simulink model "RLTunningTV"  (R2019b)
settings: Solver=odeN  StartTime=0.0  StopTime=15  FixedStep=0.001  RelTol=1e-3
PreLoadFcn:
  | Vehicle_parameters;
  | hcc_init;
InitFcn:
  | Vehicle_parameters;
  | hcc_init;
values from neighbouring files (symbols this model uses):
  c = (1.596+1.610)/2    (= 1.603)    [Vehicle_parameters.m]
  g = 9.8    [Vehicle_parameters.m]
  gamma = 0.006    [hcc_init.m]
  Jzz = 2050    [Vehicle_parameters.m]
  kx1 = 0.05890269    [hcc_init.m]
  ky1 = 0.04086363    [hcc_init.m]
  kz1 = 0.27516026    [hcc_init.m]
  lf = 1.3265    [Vehicle_parameters.m]
  lr = 1.3685    [Vehicle_parameters.m]
  M = 1360    [Vehicle_parameters.m]
  n = 6    [hcc_init.m]    (also in smoothing_t0.m = 16)
  pbk_gain = 1.0    (= 1)    [hcc_init.m]
  Q_gain = 50.0    (= 50)    [hcc_init.m]
  Qf = [0.0, 0.0 ... (first row only)    [hcc_init.m]
  Qr = [0.0, 0.0 ... (first row only)    [hcc_init.m]
  Reff = 0.323    [Vehicle_parameters.m]
  swa_gain = 45.0    (= 45)    [hcc_init.m]
  umax_m = 4000.0    (= 4000)    [hcc_init.m]
  umin_br = umin_m + umin_b    (= -4500)    [hcc_init.m]
  v = 80    [Vehicle_parameters.m]
  wFx = 0.4    [hcc_init.m]
  wFy = 0.02    [hcc_init.m]
  wGz = 1500.89459504    [hcc_init.m]
undefined symbols (not defined in the file or in its folder): DiscIntNeverNeededParam, LMUX, LMUY, sigbuilder_block
libraries: simulink x10, rllib x1
(part 1 of 3)
settings Model: Creator=st00853  LastModifiedBy=st00853
settings SolverCC: ZeroCrossControl=DisableAll
settings DebuggingCC: ArithmeticOperatorsInVariantConditions=warning
settings SFSimCC: CustomCodeUndefinedFunction=UseInterfaceOnly

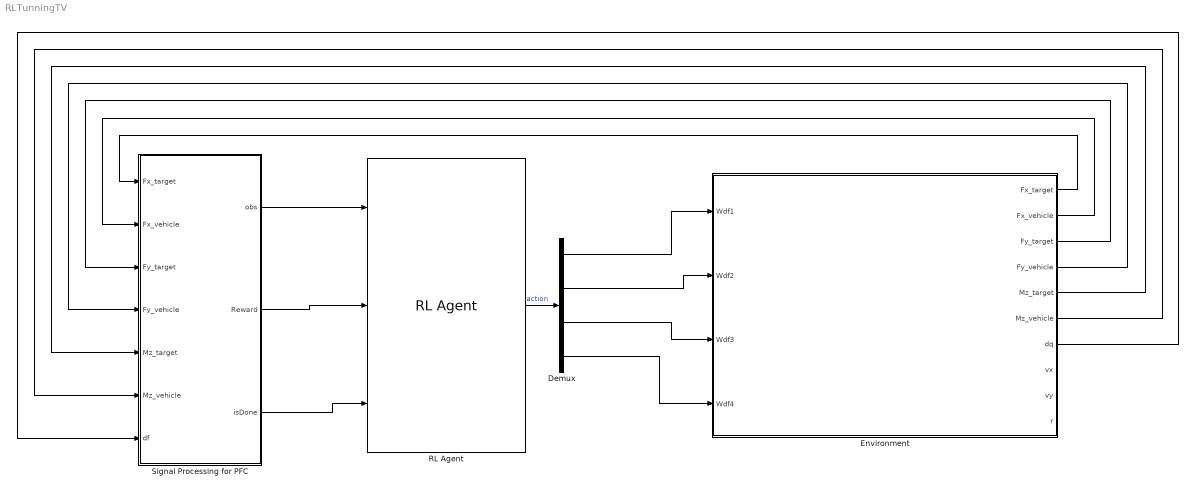
== system RLTunningTV ==
  Demux : Demux
  Environment : Subsystem
  RL Agent : rllib/RL Agent  Agent=agent  ProvideReward=on  ProvideIsDone=on  ProvideCumRwd=off  TreatAsDirectFeedthrough=on  CollectLoggedSignals=on  CollectModelStates=on
      settings: SourceProductName=Reinforcement Learning Toolbox
  Signal Processing for PFC : Subsystem
  wires:
  RL Agent/1 -> Demux/1  "action"
  Demux/1 -> Environment/1(Wdf1)
  Demux/2 -> Environment/2(Wdf2)
  Demux/3 -> Environment/3(Wdf3)
  Demux/4 -> Environment/4(Wdf4)
  Signal Processing for PFC/2(Reward) -> RL Agent/2
  Signal Processing for PFC/1(obs) -> RL Agent/1
  Signal Processing for PFC/3(isDone) -> RL Agent/3
  Environment/7(dq) -> Signal Processing for PFC/7(df)
  Environment/1(Fx_target) -> Signal Processing for PFC/1(Fx_target)
  Environment/2(Fx_vehicle) -> Signal Processing for PFC/2(Fx_vehicle)
  Environment/3(Fy_target) -> Signal Processing for PFC/3(Fy_target)
  Environment/4(Fy_vehicle) -> Signal Processing for PFC/4(Fy_vehicle)
  Environment/6(Mz_vehicle) -> Signal Processing for PFC/6(Mz_vehicle)
  Environment/5(Mz_target) -> Signal Processing for PFC/5(Mz_target)

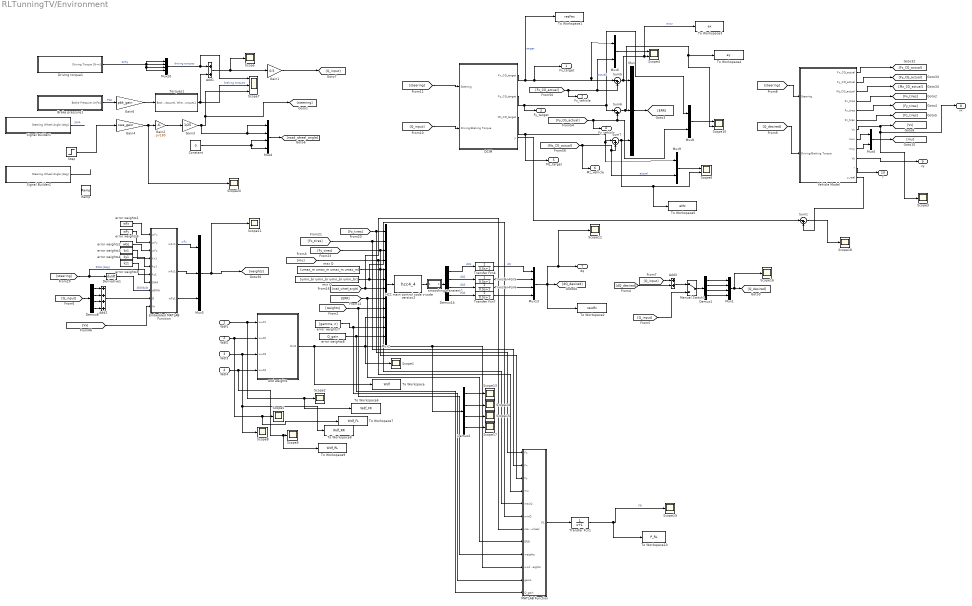
== system RLTunningTV/Environment ==
  Wdf1 : Inport
  Wdf2 : Inport  Port=2
  Wdf3 : Inport  Port=3
  Wdf4 : Inport  Port=4
  Add1 : Sum
  Add2 : Sum  Inputs=++++
  Add3 : Sum
  Brake pressure1 : Subsystem  Tag=STV Subsys  LoadFcn=sigbuilder_block('load');  StartFcn=sigbuilder_block('start');  StopFcn=sigbuilder_block('stop');  ClipboardFcn=sigbuilder_block('clipboard');  mask(Sigbuilder block){tuvar=[0:10]}
      mask help: Sigbuilder GUI
      mask init:
      | if ~strcmp(get_param(bdroot(gcbh),'SimulationStatus'),'stopped') tuvar = sigbuilder_block('maskInit'); end
      settings: CopyFcn=sigbuilder_block('copy');  DeleteFcn=sigbuilder_block('delete');  ModelCloseFcn=sigbuilder_block('modelClose');  PreSaveFcn=sigbuilder_block('preSave');  PauseFcn=sigbuilder_block('pause')  ContinueFcn=sigbuilder_block('continue')  NameChangeFcn=sigbuilder_block('namechange');  OpenFcn=sigbuilder_block('open',[0 0 1131 540.75 ]);  CloseFcn=sigbuilder_block('close');
      mask Display: plot(0, 0, 100, 100,[2, 2, 32, 32, 2], [68, 8, 8, 68, 68],[32, 2], [38, 38], [32, 19, 2],[53, 60, 44], [32, 17, 17, 2],[16, 16, 31, 31]);txt = getActiveGroup(gcbh);text(2, 100, txt,'verticalAlignment', 'top');
  Constant : Constant  Value=0
  DCIM : Subsystem
  Demux{1..2,8,14} (4 alike) : Demux
  Derivative1 : Derivative
  Driving torque1 : Subsystem  Tag=STV Subsys  LoadFcn=sigbuilder_block('load');  StartFcn=sigbuilder_block('start');  StopFcn=sigbuilder_block('stop');  ClipboardFcn=sigbuilder_block('clipboard');  mask(Sigbuilder block){tuvar=[0:10]}
      mask help: Sigbuilder GUI
      mask init:
      | if ~strcmp(get_param(bdroot(gcbh),'SimulationStatus'),'stopped') tuvar = sigbuilder_block('maskInit'); end
      settings: CopyFcn=sigbuilder_block('copy');  DeleteFcn=sigbuilder_block('delete');  ModelCloseFcn=sigbuilder_block('modelClose');  PreSaveFcn=sigbuilder_block('preSave');  PauseFcn=sigbuilder_block('pause')  ContinueFcn=sigbuilder_block('continue')  NameChangeFcn=sigbuilder_block('namechange');  OpenFcn=sigbuilder_block('open',[0 0 1131 540.75 ]);  CloseFcn=sigbuilder_block('close');
      mask Display: plot(0, 0, 100, 100,[2, 2, 32, 32, 2], [68, 8, 8, 68, 68],[32, 2], [38, 38], [32, 19, 2],[53, 60, 44], [32, 17, 17, 2],[16, 16, 31, 31]);txt = getActiveGroup(gcbh);text(2, 100, txt,'verticalAlignment', 'top');
  Embedded MATLAB Function : MATLAB Function  TreatAsAtomicUnit=on
  Gain1 : Gain  Gain=0.5  SampleTime=0.001
  Gain2 : Gain  Gain=pi/180
  Gain3 : Gain  Gain=1/25  SampleTime=0.001
  Gain4 : Gain  Gain=swa_gain  SampleTime=0.001
  Gain6 : Gain  Gain=pbk_gain  SampleTime=0.001
  HCC main control code c-code version2 : S-Function  FunctionName=hcc4_4  SFunctionDeploymentMode=off  EnableBusSupport=off
  MATLAB Function : MATLAB Function  TreatAsAtomicUnit=on
  Manual Switch1 : ManualSwitch
  Mux : Mux  Inputs=3
  Mux{1,4,13,20} (4 alike) : Mux
  Mux2 : Mux  Inputs=12
  Mux3 : Mux  Inputs=3
  Mux{5..6,8..9} (4 alike) : Mux  Inputs=2
  Ramp : simulink/Sources/Ramp  slope=0.1  start=3  InitialOutput=0
  Scope{,1..3,5,8..9,11..20} (17 alike) : Scope
  Scope10 : Scope  NumInputPorts=2
  Scope4 : Scope  NumInputPorts=2
  Scope6 : Scope  NumInputPorts=2
  Scope7 : Scope  NumInputPorts=3
  Signal Builder1 : Subsystem  Tag=STV Subsys  LoadFcn=sigbuilder_block('load');  StartFcn=sigbuilder_block('start');  StopFcn=sigbuilder_block('stop');  ClipboardFcn=sigbuilder_block('clipboard');  mask(Sigbuilder block){tuvar=[0:10]}
      mask help: Sigbuilder GUI
      mask init:
      | if ~strcmp(get_param(bdroot(gcbh),'SimulationStatus'),'stopped') tuvar = sigbuilder_block('maskInit'); end
      settings: CopyFcn=sigbuilder_block('copy');  DeleteFcn=sigbuilder_block('delete');  ModelCloseFcn=sigbuilder_block('modelClose');  PreSaveFcn=sigbuilder_block('preSave');  PauseFcn=sigbuilder_block('pause')  ContinueFcn=sigbuilder_block('continue')  NameChangeFcn=sigbuilder_block('namechange');  OpenFcn=sigbuilder_block('open',[96.75 77.25 1131 540.75 ]);  CloseFcn=sigbuilder_block('close');
      mask Display: plot(0, 0, 100, 100,[2, 2, 32, 32, 2], [68, 8, 8, 68, 68],[32, 2], [38, 38], [32, 19, 2],[53, 60, 44], [32, 17, 17, 2],[16, 16, 31, 31]);txt = getActiveGroup(gcbh);text(2, 100, txt,'verticalAlignment', 'top');
  Signal Builder2 : Subsystem  Tag=STV Subsys  LoadFcn=sigbuilder_block('load');  StartFcn=sigbuilder_block('start');  StopFcn=sigbuilder_block('stop');  ClipboardFcn=sigbuilder_block('clipboard');  mask(Sigbuilder block){tuvar=[0:10]}
      mask help: Sigbuilder GUI
      mask init:
      | if ~strcmp(get_param(bdroot(gcbh),'SimulationStatus'),'stopped') tuvar = sigbuilder_block('maskInit'); end
      settings: CopyFcn=sigbuilder_block('copy');  DeleteFcn=sigbuilder_block('delete');  ModelCloseFcn=sigbuilder_block('modelClose');  PreSaveFcn=sigbuilder_block('preSave');  PauseFcn=sigbuilder_block('pause')  ContinueFcn=sigbuilder_block('continue')  NameChangeFcn=sigbuilder_block('namechange');  OpenFcn=sigbuilder_block('open',[111 159.75 1131 540.75 ]);  CloseFcn=sigbuilder_block('close');
      mask Display: plot(0, 0, 100, 100,[2, 2, 32, 32, 2], [68, 8, 8, 68, 68],[32, 2], [38, 38], [32, 19, 2],[53, 60, 44], [32, 17, 17, 2],[16, 16, 31, 31]);txt = getActiveGroup(gcbh);text(2, 100, txt,'verticalAlignment', 'top');
  Step : Step  Time=3.5  SampleTime=0.001
  Sum{1,5..7} (4 alike) : Sum  Inputs=|-+
  To Workspace : ToWorkspace  VariableName=Wdf  SaveFormat=Structure With Time  SampleTime=-1
  To Workspace1 : ToWorkspace  VariableName=resFex  SaveFormat=Structure With Time  SampleTime=-1
  To Workspace10 : ToWorkspace  VariableName=P_RL  SaveFormat=Structure With Time  SampleTime=-1
  To Workspace2 : ToWorkspace  VariableName=resdfx  SaveFormat=Structure With Time  SampleTime=-1
  To Workspace3 : ToWorkspace  VariableName=ex  SaveFormat=Structure With Time  SampleTime=-1
  To Workspace4 : ToWorkspace  VariableName=ey  SaveFormat=Structure With Time  SampleTime=-1
  To Workspace5 : ToWorkspace  VariableName=eMz  SaveFormat=Structure With Time  SampleTime=-1
  To Workspace6 : ToWorkspace  VariableName=Wdf_FR  SaveFormat=Structure With Time  SampleTime=-1
  To Workspace7 : ToWorkspace  VariableName=Wdf_FL  SaveFormat=Structure With Time  SampleTime=-1
  To Workspace8 : ToWorkspace  VariableName=Wdf_RR  SaveFormat=Structure With Time  SampleTime=-1
  To Workspace9 : ToWorkspace  VariableName=Wdf_RL  SaveFormat=Structure With Time  SampleTime=-1
  Torques1 : Subsystem
  Transfer Fcn1 : TransferFcn  Denominator=[1 1]
  Transfer Fcn{4..7} (4 alike) : TransferFcn  Denominator=[0.5 1]
  Vehicle Model : Subsystem
  error weights1 : Constant  Value=wFx
  error weights2 : Constant  Value=wGz
  error weights3 : Constant  Value=kx1
  error weights4 : Constant  Value=ky1
  error weights5 : Constant  Value=kz1
  error weights6 : Constant  Value=wFy
  error weights7 : Constant  Value=[gamma, n]
  error weights8 : Constant  Value=Q_gain
  max Q : Constant  Value=[umax_m umax_m umax_m umax_m]
  min Q : Constant  Value=[umin_br umin_br umin_br umin_br]
  smoothing transient2 : Subsystem
  wxd weights : Subsystem
  Fx_target : Outport
  Fx_vehicle : Outport  Port=2
  Fy_target : Outport  Port=3
  Fy_vehicle : Outport  Port=4
  Mz_target : Outport  Port=5
  Mz_vehicle : Outport  Port=6
  dq : Outport  Port=7
  vx : Outport  Port=8
  vy : Outport  Port=9
  r : Outport  Port=10
  wires:
  Demux1/3 -> Mux1/3
  Transfer Fcn6/1 -> Mux13/3
  Demux1/4 -> Mux1/4
  Vehicle Model/8(mux) -> Mux5/1
  Constant/1 -> Mux4/4, Mux4/3
  error weights3/1 -> Embedded MATLAB Function/4(kx1)
  Embedded MATLAB Function/1(wFx1) -> Mux3/1  "wFx"
  max Q/1 -> MATLAB Function/5(maxQ), Mux2/5
  Vehicle Model/3("Mz_CG_actual ") -> [Mz_CG_actual]
  [ERR] -> MATLAB Function/8(ERR), Mux2/8
  Gain6/1 -> Torques1/1(Brake pressure1)
  Vehicle Model/9(muy) -> Mux5/2
  Demux14/2 -> Transfer Fcn5/1  "dQ2"
  Vehicle Model/6(Fz_tires) -> [Fz_tires]
  [Q_input] -> Demux8/1
  [Q_input] -> Add3/1
  error weights5/1 -> Embedded MATLAB Function/6(kz1)
  DCIM/1(Fx_CG_target) -> To Workspace1/1, Fx_target/1, Mux6/1, Sum5/1  "target"
  Demux8/1 -> Add2/1
  Vehicle Model/4(Fx_tires) -> [Fx_tires]
  [weights] -> MATLAB Function/9(weights), Mux2/9
  Derivative1/1 -> Embedded MATLAB Function/8(dSWA)  "dSWA/dt"
  [Q_input] -> Manual Switch1/2
  Driving torque1/1(Driving Torque [N-m]) -> Mux20/4, Mux20/3, Mux20/2, Mux20/1  "DrTq"
  Demux1/1 -> Mux1/1
  Mux20/1 -> Scope7/1, Add1/1  "driving torques"
  Mux2/1 -> HCC main control code c-code version2/1
  Brake pressure1/1(Brake Pressure [mPa]) -> Gain6/1  "PbK"
  [dQ_desired] -> Add3/2
  Demux14/3 -> Transfer Fcn6/1  "dQ3"
  Demux1/2 -> Mux1/2
  Vehicle Model/5(Fy_tires) -> [Fy_tires]
  [steering] -> Embedded MATLAB Function/7(SWA), Derivative1/1  "SWA [deg]"
  Signal Builder1/1(Steering Wheel Angle [deg]) -> ?  "SWA"
  [Fx_CG_actual] -> Fx_vehicle/1, Mux6/2, Sum5/2  "actual"
  [Fz_tires] -> MATLAB Function/1(Fz), Mux2/1
  Manual Switch1/1 -> Demux1/1
  [Vx] -> Embedded MATLAB Function/10(Vx)
  Vehicle Model/7(Vx) -> [Vx], Scope3/1, vx/1
  Embedded MATLAB Function/2(wFy1) -> Mux3/2
  Transfer Fcn4/1 -> Mux13/1  "dQ"
  Vehicle Model/1(Fx_CG_actual) -> [Fx_CG_actual]
  error weights2/1 -> Embedded MATLAB Function/3(wFz)
  [Q_input] -> DCIM/2(Driving/Braking Torque)
  error weights4/1 -> Embedded MATLAB Function/5(ky1)
  error weights7/1 -> MATLAB Function/11(gains), Mux2/11
  Add3/1 -> Manual Switch1/1
  wxd weights/1(Out1) -> To Workspace/1, MATLAB Function/10(wxd_weights), Demux2/1, Mux2/10, Scope1/1
  Gain3/1 -> Mux4/2, Mux4/1, [steering], Scope7/3
  [mu] -> MATLAB Function/4(mu), Mux2/4
  min Q/1 -> MATLAB Function/6(minQ), Mux2/6
  Demux14/1 -> Transfer Fcn4/1  "dQ1"
  Transfer Fcn7/1 -> Mux13/4
  Mux5/1 -> [mu]
  Demux14/4 -> Transfer Fcn7/1  "dQ4"
  Demux8/4 -> Add2/4
  Mux4/1 -> [road_wheel_angle]
  Mux13/1 -> To Workspace2/1, Scope12/1, dq/1, [dQ_desired]
  Add2/1 -> Embedded MATLAB Function/9(Q)
  Vehicle Model/2("Fy_CG_actual ") -> [Fy_CG_actual]
  Demux8/3 -> Add2/3
  Torques1/1(Wheel torques1) -> Scope7/2, Add1/2  "braking torques"
  [Fy_tires] -> MATLAB Function/3(Fy), Mux2/3
  Mux9/1 -> Scope6/1
  Gain4/1 -> Scope20/1, Gain2/1
  [Q_desired] -> Vehicle Model/2(Driving/Braking Torque)
  HCC main control code c-code version2/1 -> smoothing transient2/1(In1)
  Gain1/1 -> [Q_input]
  Demux8/2 -> Add2/2
  Sum5/1 -> To Workspace3/1, Scope4/2, Mux/1  "error"
  Gain2/1 -> Gain3/1
  Sum6/1 -> Mux/2, Scope10/2, To Workspace4/1
  DCIM/2("Fy_CG_target ") -> Fy_target/1, Sum6/1, Mux8/1
  error weights8/1 -> MATLAB Function/12(Q_gain), Mux2/12
  Embedded MATLAB Function/3(wFz1) -> Mux3/3
  Sum7/1 -> Mux/3, To Workspace5/1, Scope6/2
  [Fy_CG_actual] -> Fy_vehicle/1, Mux8/2, Sum6/2
  Transfer Fcn5/1 -> Mux13/2
  [road_wheel_angle] -> Mux2/7, MATLAB Function/7(road_wheel)
  Mux6/1 -> Scope4/1
  [steering] -> Vehicle Model/1(Steering)
  DCIM/3("Mz_CG_target ") -> Mz_target/1, Mux9/1, Sum7/1
  Add1/1 -> Scope/1, Gain1/1
  [Mz_CG_actual] -> Mz_vehicle/1, Mux9/2, Sum7/2  "actual"
  Mux/1 -> [ERR]
  Mux3/1 -> Scope11/1, [weights]
  Mux8/1 -> Scope10/1
  Mux1/1 -> Scope16/1, [Q_desired]
  [steering] -> DCIM/1(Steering)
  smoothing transient2/1(Out1) -> Demux14/1
  [Fx_tires] -> MATLAB Function/2(Fx), Mux2/2
  Wdf2/1 -> To Workspace7/1, Scope5/1, wxd weights/2(wxd2)
  Wdf3/1 -> Scope8/1, To Workspace8/1, wxd weights/3(wxd3)
  Wdf4/1 -> To Workspace9/1, Scope9/1, wxd weights/4(wxd4)
  Vehicle Model/10(Vy) -> vy/1
  Vehicle Model/11(r) -> r/1
  error weights1/1 -> Embedded MATLAB Function/1(wFx)
  error weights6/1 -> Embedded MATLAB Function/2(wFy)
  Wdf1/1 -> To Workspace6/1, Scope2/1, wxd weights/1(wxd1)
  Demux2/1 -> Scope13/1
  Demux2/2 -> Scope14/1
  Demux2/3 -> Scope15/1
  Demux2/4 -> Scope17/1
  DCIM/4(y) -> Sum1/1
  Vehicle Model/12(y_real) -> Sum1/2
  Sum1/1 -> Scope18/1
  MATLAB Function/1(P1) -> Transfer Fcn1/1
  Transfer Fcn1/1 -> To Workspace10/1, Scope19/1  "FR"
  Signal Builder2/1(Steering Wheel Angle [deg]) -> ?
  Step/1 -> Gain4/1

== system RLTunningTV/Signal Processing for PFC ==
  Fx_target : Inport
  Fx_vehicle : Inport  Port=2
  Fy_target : Inport  Port=3
  Fy_vehicle : Inport  Port=4
  Mz_target : Inport  Port=5
  Mz_vehicle : Inport  Port=6
  df : Inport  Port=7
  Subsystem : Subsystem
  Subsystem1 : Subsystem
  Subsystem2 : Subsystem
  obs : Outport  VectorParamsAs1DForOutWhenUnconnected=off
  Reward : Outport  Port=2  VectorParamsAs1DForOutWhenUnconnected=off
  isDone : Outport  Port=3  VectorParamsAs1DForOutWhenUnconnected=off
  wires:
  Subsystem/1(obs) -> obs/1
  Subsystem2/1(isDone) -> isDone/1
  Fx_target/1 -> Subsystem/1(Fx_target)
  Fx_vehicle/1 -> Subsystem/2(Fx_vehicle)
  Fy_target/1 -> Subsystem/4(Fy_target)
  Fy_vehicle/1 -> Subsystem/3(Fy_vehicle)
  Mz_vehicle/1 -> Subsystem/5(Mz_vehicle)
  Mz_target/1 -> Subsystem/6(Mz_target)
  df/1 -> Subsystem/7(df)
  Subsystem/2(ex) -> Subsystem2/1(ex), Subsystem1/2(ex)
  Subsystem/3(ey) -> Subsystem2/2(ey), Subsystem1/1(ey)
  Subsystem/4(Mz) -> Subsystem2/3(Mz), Subsystem1/3(Mz)
  Subsystem1/1(reward) -> Reward/1

== system RLTunningTV/Environment/Brake pressure1 ==
  Demux : Demux  Tag=STV Demux  Outputs=1
  FromWs : FromWorkspace  Tag=STV FromWs  VariableName=tuvar  SampleTime=0
      SigBuilderData=|
      | common.afterFinalStr = 'Extrapolate'
      | common.sampleTime = 0
      | dataSet.timeRange = [0 15]
      | dataSet.name = 'Group 1'
      | sbobj.Groups.Name = 'Group 1'
      | sbobj.Groups.Signals.Name = 'Brake Pressure [mPa]'
      | sbobj.Groups.Signals.XData = [0 2 3.3 5 5.3 8 8.5 9.5 10 10 15]
      | sbobj.Groups.Signals.YData = [0 0 2 2 0 0 4.05 4.05 -0.1 0 -0.05]
      | sbobj.Groups.TimeRange = [0 15]
  Brake Pressure [mPa] : Outport  Tag=STV Outport  VectorParamsAs1DForOutWhenUnconnected=off
  wires:
  FromWs/1 -> Demux/1
  Demux/1 -> Brake Pressure [mPa]/1

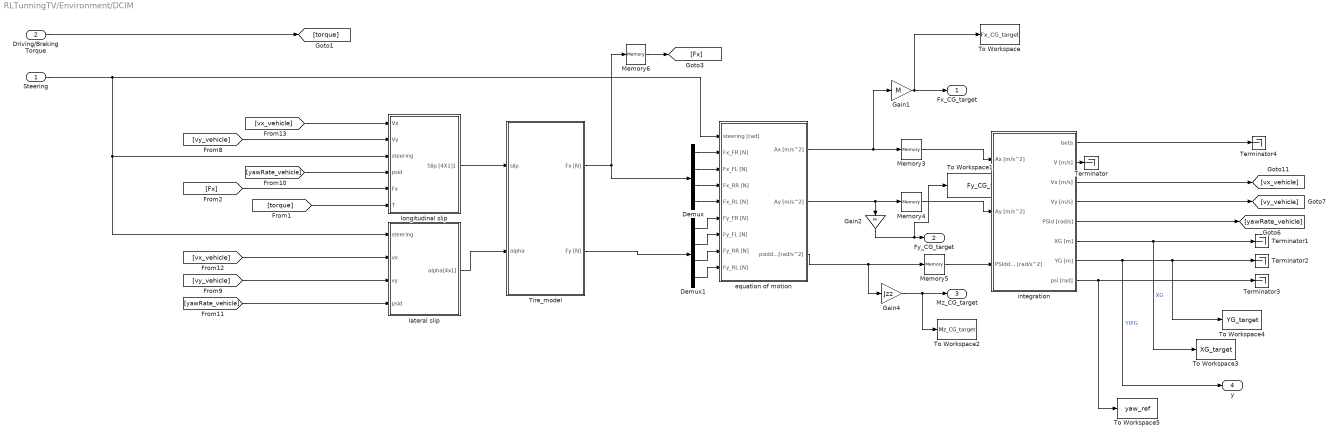
== system RLTunningTV/Environment/DCIM ==
  Steering : Inport
  Driving/Braking Torque : Inport  Port=2
  Demux : Demux
  Demux1 : Demux
  Gain1 : Gain  Gain=M
  Gain2 : Gain  Gain=M
  Gain4 : Gain  Gain=Jzz
  Memory{3..6} (4 alike) : Memory
  Terminator{,1..4} (5 alike) : Terminator
  Tire_model : Subsystem  TreatAsAtomicUnit=on
  To Workspace : ToWorkspace  VariableName=Fx_CG_target  SaveFormat=Structure With Time  SampleTime=-1
  To Workspace1 : ToWorkspace  VariableName=Fy_CG_target  SaveFormat=Structure With Time  SampleTime=-1
  To Workspace2 : ToWorkspace  VariableName=Mz_CG_target  SaveFormat=Structure With Time  SampleTime=-1
  To Workspace3 : ToWorkspace  VariableName=XG_target  SaveFormat=Structure With Time  SampleTime=-1
  To Workspace4 : ToWorkspace  VariableName=YG_target  SaveFormat=Structure With Time  SampleTime=-1
  To Workspace5 : ToWorkspace  VariableName=yaw_ref  SaveFormat=Structure With Time  SampleTime=-1
  equation of motion : Subsystem  TreatAsAtomicUnit=on
  integration : Subsystem  TreatAsAtomicUnit=on
  lateral slip : Subsystem  TreatAsAtomicUnit=on
  longitudinal slip : Subsystem  TreatAsAtomicUnit=on
  Fx_CG_target : Outport  VectorParamsAs1DForOutWhenUnconnected=off
  "Fy_CG_target " : Outport  Port=2  VectorParamsAs1DForOutWhenUnconnected=off
  "Mz_CG_target " : Outport  Port=3  VectorParamsAs1DForOutWhenUnconnected=off
  y : Outport  Port=4  VectorParamsAs1DForOutWhenUnconnected=off
  wires:
  Gain2/1 -> To Workspace1/1, "Fy_CG_target "/1
  Steering/1 -> lateral slip/1(steering), longitudinal slip/3(steering), equation of motion/1(steering [rad])
  Memory5/1 -> integration/3(PSIddot [rad/s^2])
  Tire_model/2(Fy [N]) -> Demux1/1
  [vx_vehicle] -> longitudinal slip/1(Vx)
  Demux1/3 -> equation of motion/8(Fy_RR [N])
  [torque] -> longitudinal slip/6(T)
  [yawRate_vehicle] -> longitudinal slip/4(psid)
  Memory4/1 -> integration/2(Ay [m/s^2])
  Memory3/1 -> integration/1(Ax [m/s^2])
  equation of motion/3(psiddot [rad/s^2]) -> Memory5/1, Gain4/1
  Demux/2 -> equation of motion/3(Fx_FL [N])
  integration/8(psi [rad]) -> To Workspace5/1, Terminator3/1
  integration/2(V [m/s]) -> Terminator/1
  Tire_model/1(Fx [N]) -> Demux/1, Memory6/1
  equation of motion/1(Ax [m/s^2]) -> Gain1/1, Memory3/1
  Driving/Braking Torque/1 -> [torque]
  Demux/3 -> equation of motion/4(Fx_RR [N])
  Demux/4 -> equation of motion/5(Fx_RL [N])
  equation of motion/2(Ay [m/s^2]) -> Memory4/1, Gain2/1
  integration/7(YG [m]) -> y/1, To Workspace4/1, Terminator2/1  "YIPG"
  integration/1(beta) -> Terminator4/1
  integration/6(XG [m]) -> To Workspace3/1, Terminator1/1  "XG"
  Memory6/1 -> [Fx]
  Demux1/1 -> equation of motion/6(Fy_FR [N])
  Demux1/2 -> equation of motion/7(Fy_FL [N])
  [vy_vehicle] -> lateral slip/3(vy)
  [Fx] -> longitudinal slip/5(Fx)
  Demux/1 -> equation of motion/2(Fx_FR [N])
  lateral slip/1(alpha[4x1]) -> Tire_model/2(alpha)
  Gain4/1 -> To Workspace2/1, "Mz_CG_target "/1
  Demux1/4 -> equation of motion/9(Fy_RL [N])
  longitudinal slip/1(Slip [4X1]1) -> Tire_model/1("slip ")
  [vy_vehicle] -> longitudinal slip/2(Vy)
  integration/5(PSId [rad/s]) -> [yawRate_vehicle]
  integration/4(Vy [m/s]) -> [vy_vehicle]
  [vx_vehicle] -> lateral slip/2(vx)
  integration/3(Vx [m/s]) -> [vx_vehicle]
  [yawRate_vehicle] -> lateral slip/4(psid)
  Gain1/1 -> To Workspace/1, Fx_CG_target/1

== system RLTunningTV/Environment/Driving torque1 ==
  Demux : Demux  Tag=STV Demux  Outputs=1
  FromWs : FromWorkspace  Tag=STV FromWs  VariableName=tuvar  SampleTime=0
      SigBuilderData=|
      | common.afterFinalStr = 'Extrapolate'
      | common.sampleTime = 0
      | dataSet.timeRange = [0 15]
      | dataSet.name = 'Group 1'
      | sbobj.Groups.Name = 'Group 1'
      | sbobj.Groups.Signals.Name = 'Driving Torque [N-m]'
      | sbobj.Groups.Signals.XData = [0 2.5 4 7 8.5 9 10 12 13 15]
      | sbobj.Groups.Signals.YData = [0 0 0 0 0 0 0 890 900 -70]
      | sbobj.Groups.TimeRange = [0 15]
  Driving Torque [N-m] : Outport  Tag=STV Outport  VectorParamsAs1DForOutWhenUnconnected=off
  wires:
  FromWs/1 -> Demux/1
  Demux/1 -> Driving Torque [N-m]/1

== system RLTunningTV/Environment/Signal Builder1 ==
  Demux : Demux  Tag=STV Demux  Outputs=1
  FromWs : FromWorkspace  Tag=STV FromWs  VariableName=tuvar  SampleTime=0
      SigBuilderData=|
      | common.afterFinalStr = 'Extrapolate'
      | common.sampleTime = 0
      | dataSet.timeRange = [0 15]
      | dataSet.name = 'Group 1'
      | sbobj.Groups.Name = 'Group 1'
      | sbobj.Groups.Signals.Name = 'Steering Wheel Angle [deg]'
      | sbobj.Groups.Signals.XData = [0 0.5 1 1.5 2 2.5 3 3.5 4.5 5 5.5 6 6.2 6.5 7 10 15]
      | sbobj.Groups.Signals.YData = [0 0 1 0.99 -1 -1 0.99 0.98 -0.99 -1 0.63 0.63 -0.69 -0.68 0.07 -0.09 0.06]
      | sbobj.Groups.TimeRange = [0 15]
  Steering Wheel Angle [deg] : Outport  Tag=STV Outport  VectorParamsAs1DForOutWhenUnconnected=off
  wires:
  Demux/1 -> Steering Wheel Angle [deg]/1
  FromWs/1 -> Demux/1

== system RLTunningTV/Environment/Signal Builder2 ==
  Demux : Demux  Tag=STV Demux  Outputs=1
  FromWs : FromWorkspace  Tag=STV FromWs  VariableName=tuvar  SampleTime=0
      SigBuilderData=|
      | common.afterFinalStr = 'Extrapolate'
      | common.sampleTime = 0
      | dataSet.timeRange = [0 15]
      | dataSet.name = 'Group 1'
      | sbobj.Groups.Name = 'Group 1'
      | sbobj.Groups.Signals.Name = 'Steering Wheel Angle [deg]'
      | sbobj.Groups.Signals.XData = [0 0.5 1 1.5 2 2.5 3 3.5 4.5 5 5.5 6 6.2 6.5 7 10 15]
      | sbobj.Groups.Signals.YData = [0 0 0.9 0.9 0.9 0.9 0.9 0.9 0.9 0.9 0 -0.9 -0.9 -0.9 -0.9 -0.9 0.01]
      | sbobj.Groups.TimeRange = [0 15]
  Steering Wheel Angle [deg] : Outport  Tag=STV Outport  VectorParamsAs1DForOutWhenUnconnected=off
  wires:
  FromWs/1 -> Demux/1
  Demux/1 -> Steering Wheel Angle [deg]/1

== system RLTunningTV/Environment/Torques1 ==
  Brake pressure1 : Inport
  1-D Lookup Table : Lookup_n-D  NumberOfTableDimensions=1  BreakpointsForDimension1=Qf(:,1)  Table=-Qf(:,2)  InternalRulePriority=Speed  RndMeth=Simplest  InputSameDT=on
  1-D Lookup Table1 : Lookup_n-D  NumberOfTableDimensions=1  BreakpointsForDimension1=Qf(:,1)  Table=-Qf(:,2)  InternalRulePriority=Speed  RndMeth=Simplest  InputSameDT=on
  1-D Lookup Table2 : Lookup_n-D  NumberOfTableDimensions=1  BreakpointsForDimension1=Qr(:,1)  Table=-Qr(:,2)  InternalRulePriority=Speed  RndMeth=Simplest  InputSameDT=on
  1-D Lookup Table3 : Lookup_n-D  NumberOfTableDimensions=1  BreakpointsForDimension1=Qr(:,1)  Table=-Qr(:,2)  InternalRulePriority=Speed  RndMeth=Simplest  InputSameDT=on
  Mux1 : Mux
  Mux2 : Mux  Inputs=2
  Scope1 : Scope
  Transfer Fcn LF1 : TransferFcn  Denominator=[0.06 1]
  Wheel torques1 : Outport  VectorParamsAs1DForOutWhenUnconnected=off
  wires:
  1-D Lookup Table3/1 -> Mux1/4
  Mux1/1 -> Wheel torques1/1
  Brake pressure1/1 -> Mux2/2, Transfer Fcn LF1/1
  Transfer Fcn LF1/1 -> Mux2/1, 1-D Lookup Table2/1, 1-D Lookup Table3/1, 1-D Lookup Table1/1, 1-D Lookup Table/1
  Mux2/1 -> Scope1/1
  1-D Lookup Table2/1 -> Mux1/3
  1-D Lookup Table1/1 -> Mux1/2
  1-D Lookup Table/1 -> Mux1/1

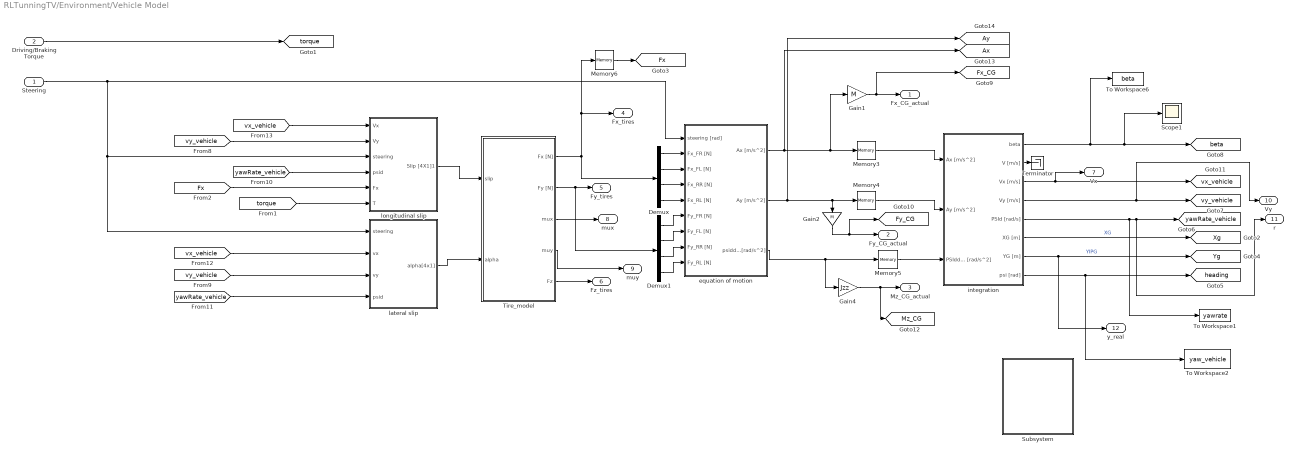
== system RLTunningTV/Environment/Vehicle Model ==
  Steering : Inport
  Driving/Braking Torque : Inport  Port=2
  Demux : Demux
  Demux1 : Demux
  Gain1 : Gain  Gain=M
  Gain2 : Gain  Gain=M
  Gain4 : Gain  Gain=Jzz
  Memory{3..6} (4 alike) : Memory
  Scope1 : Scope
  Subsystem : Subsystem
  Terminator : Terminator
  Tire_model : Subsystem  TreatAsAtomicUnit=on
  To Workspace1 : ToWorkspace  VariableName=yawrate  SaveFormat=Structure With Time  SampleTime=-1
  To Workspace2 : ToWorkspace  VariableName=yaw_vehicle  SaveFormat=Structure With Time  SampleTime=-1
  To Workspace6 : ToWorkspace  VariableName=beta  SaveFormat=Structure With Time  SampleTime=-1
  equation of motion : Subsystem  TreatAsAtomicUnit=on
  integration : Subsystem  TreatAsAtomicUnit=on
  lateral slip : Subsystem  TreatAsAtomicUnit=on
  longitudinal slip : Subsystem  TreatAsAtomicUnit=on
  Fx_CG_actual : Outport  VectorParamsAs1DForOutWhenUnconnected=off
  "Fy_CG_actual " : Outport  Port=2  VectorParamsAs1DForOutWhenUnconnected=off
  "Mz_CG_actual " : Outport  Port=3  VectorParamsAs1DForOutWhenUnconnected=off
  Fx_tires : Outport  Port=4  VectorParamsAs1DForOutWhenUnconnected=off
  Fy_tires : Outport  Port=5  VectorParamsAs1DForOutWhenUnconnected=off
  Fz_tires : Outport  Port=6  VectorParamsAs1DForOutWhenUnconnected=off
  Vx : Outport  Port=7  VectorParamsAs1DForOutWhenUnconnected=off
  mux : Outport  Port=8  VectorParamsAs1DForOutWhenUnconnected=off
  muy : Outport  Port=9  VectorParamsAs1DForOutWhenUnconnected=off
  Vy : Outport  Port=10  VectorParamsAs1DForOutWhenUnconnected=off
  r : Outport  Port=11  VectorParamsAs1DForOutWhenUnconnected=off
  y_real : Outport  Port=12  VectorParamsAs1DForOutWhenUnconnected=off
  tag scope: Ax=global, Ay=global, Fx=global, Fx_CG=global, Fy_CG=global, Mz_CG=global, Xg=global, Yg=global, beta=global, heading=global, torque=global, vx_vehicle=global, vy_vehicle=global, yawRate_vehicle=global
  wires:
  [yawRate_vehicle] -> lateral slip/4(psid)
  integration/3(Vx [m/s]) -> Vx/1, [vx_vehicle]
  [vx_vehicle] -> lateral slip/2(vx)
  integration/4(Vy [m/s]) -> Vy/1, [vy_vehicle]
  [vy_vehicle] -> longitudinal slip/2(Vy)
  longitudinal slip/1(Slip [4X1]1) -> Tire_model/1("slip ")
  Demux1/4 -> equation of motion/9(Fy_RL [N])
  Gain4/1 -> [Mz_CG], "Mz_CG_actual "/1
  lateral slip/1(alpha[4x1]) -> Tire_model/2(alpha)
  Demux/1 -> equation of motion/2(Fx_FR [N])
  [Fx] -> longitudinal slip/5(Fx)
  [vy_vehicle] -> lateral slip/3(vy)
  Demux1/2 -> equation of motion/7(Fy_FL [N])
  Demux1/1 -> equation of motion/6(Fy_FR [N])
  Memory6/1 -> [Fx]
  integration/6(XG [m]) -> [Xg]  "XG"
  integration/7(YG [m]) -> y_real/1, [Yg]  "YIPG"
  equation of motion/2(Ay [m/s^2]) -> [Ay], Gain2/1, Memory4/1
  Demux/4 -> equation of motion/5(Fx_RL [N])
  Tire_model/3(mux) -> mux/1
  Demux/3 -> equation of motion/4(Fx_RR [N])
  Driving/Braking Torque/1 -> [torque]
  equation of motion/1(Ax [m/s^2]) -> [Ax], Memory3/1, Gain1/1
  Tire_model/1(Fx [N]) -> Fx_tires/1, Memory6/1, Demux/1
  integration/2(V [m/s]) -> Terminator/1
  integration/8(psi [rad]) -> To Workspace2/1, [heading]
  Demux/2 -> equation of motion/3(Fx_FL [N])
  equation of motion/3(psiddot [rad/s^2]) -> Gain4/1, Memory5/1
  Memory3/1 -> integration/1(Ax [m/s^2])
  Memory4/1 -> integration/2(Ay [m/s^2])
  [yawRate_vehicle] -> longitudinal slip/4(psid)
  [torque] -> longitudinal slip/6(T)
  Demux1/3 -> equation of motion/8(Fy_RR [N])
  [vx_vehicle] -> longitudinal slip/1(Vx)
  Gain1/1 -> [Fx_CG], Fx_CG_actual/1
  Tire_model/4(muy) -> muy/1
  Tire_model/2(Fy [N]) -> Demux1/1, Fy_tires/1
  Memory5/1 -> integration/3(PSIddot [rad/s^2])
  Tire_model/5(Fz) -> Fz_tires/1
  Steering/1 -> equation of motion/1(steering [rad]), longitudinal slip/3(steering), lateral slip/1(steering)
  Gain2/1 -> [Fy_CG], "Fy_CG_actual "/1
  integration/5(PSId [rad/s]) -> To Workspace1/1, r/1, [yawRate_vehicle]
  integration/1(beta) -> To Workspace6/1, Scope1/1, [beta]

== system RLTunningTV/Environment/smoothing transient2 ==
  In1 : Inport
  Clock : Clock
  MATLAB Fcn : MATLABFcn  MATLABFcn=smoothing_t0
  Product2 : Product  RndMeth=Zero
  Out1 : Outport  VectorParamsAs1DForOutWhenUnconnected=off
  wires:
  In1/1 -> Product2/2
  Product2/1 -> Out1/1
  Clock/1 -> MATLAB Fcn/1
  MATLAB Fcn/1 -> Product2/1

== system RLTunningTV/Environment/wxd weights ==
  wxd1 : Inport
  wxd2 : Inport  Port=2
  wxd3 : Inport  Port=3
  wxd4 : Inport  Port=4
  Demux8 : Demux
  Mux17 : Mux
  Product{1..8} (8 alike) : Product  RndMeth=Zero
  error weights5 : Constant  Value=[1.0 1.0 1.0 1.0]'
  failure{1..4} (4 alike) : Step  Time=4  Before=1  SampleTime=0
  Out1 : Outport  VectorParamsAs1DForOutWhenUnconnected=off
  wires:
  Mux17/1 -> Out1/1
  Product8/1 -> Mux17/4
  Product7/1 -> Mux17/3
  Product6/1 -> Mux17/2
  Product5/1 -> Mux17/1
  Demux8/4 -> Product4/2
  Demux8/3 -> Product3/2
  Demux8/2 -> Product1/2
  Demux8/1 -> Product2/2
  error weights5/1 -> Demux8/1
  Product4/1 -> Product8/1
  wxd4/1 -> Product4/1
  Product3/1 -> Product7/1
  wxd3/1 -> Product3/1
  Product1/1 -> Product6/1
  wxd2/1 -> Product1/1
  wxd1/1 -> Product2/1
  Product2/1 -> Product5/1
  failure4/1 -> Product8/2
  failure3/1 -> Product7/2
  failure2/1 -> Product6/2
  failure1/1 -> Product5/2

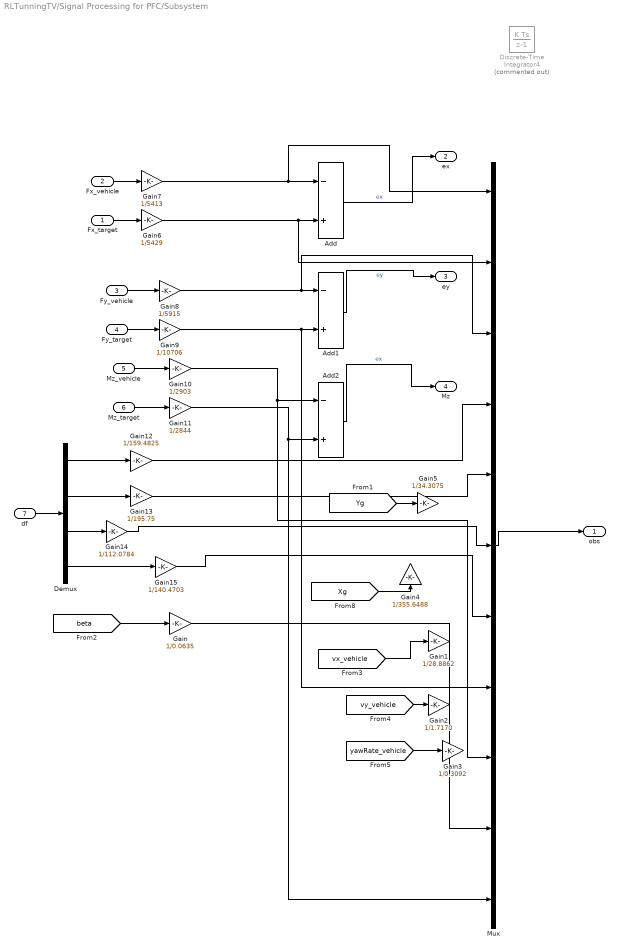
== system RLTunningTV/Signal Processing for PFC/Subsystem ==
  Fx_target : Inport
  Fx_vehicle : Inport  Port=2
  Fy_vehicle : Inport  Port=3
  Fy_target : Inport  Port=4
  Mz_vehicle : Inport  Port=5
  Mz_target : Inport  Port=6
  df : Inport  Port=7
  Add : Sum  Inputs=-+
  Add1 : Sum  Inputs=-+
  Add2 : Sum  Inputs=-+
  Demux : Demux
  Discrete-Time Integrator4 : DiscreteIntegrator  Commented=on  SampleTime=-1  ICPrevOutput=DiscIntNeverNeededParam  ICPrevScaledInput=DiscIntNeverNeededParam
  Gain : Gain  Gain=1/0.0635
  Gain1 : Gain  Gain=1/28.8862
  Gain10 : Gain  Gain=1/2903
  Gain11 : Gain  Gain=1/2844
  Gain12 : Gain  Gain=1/159.4825
  Gain13 : Gain  Gain=1/195.75
  Gain14 : Gain  Gain=1/112.0784
  Gain15 : Gain  Gain=1/140.4703
  Gain2 : Gain  Gain=1/1.7170
  Gain3 : Gain  Gain=1/0.3092
  Gain4 : Gain  Gain=1/355.6488
  Gain5 : Gain  Gain=1/34.3075
  Gain6 : Gain  Gain=1/5429
  Gain7 : Gain  Gain=1/5413
  Gain8 : Gain  Gain=1/5915
  Gain9 : Gain  Gain=1/10706
  Mux : Mux  Inputs=11
  obs : Outport  VectorParamsAs1DForOutWhenUnconnected=off
  ex : Outport  Port=2  VectorParamsAs1DForOutWhenUnconnected=off
  ey : Outport  Port=3  VectorParamsAs1DForOutWhenUnconnected=off
  Mz : Outport  Port=4  VectorParamsAs1DForOutWhenUnconnected=off
  wires:
  Fx_target/1 -> Gain6/1
  Mux/1 -> obs/1
  Fx_vehicle/1 -> Gain7/1
  Add/1 -> ex/1  "ex"
  Fy_vehicle/1 -> Gain8/1
  Fy_target/1 -> Gain9/1
  Add1/1 -> ey/1  "ey"
  Add2/1 -> Mz/1  "ex"
  Mz_vehicle/1 -> Gain10/1
  Mz_target/1 -> Gain11/1
  df/1 -> Demux/1
  Demux/1 -> Gain12/1
  Demux/2 -> Gain13/1
  Demux/3 -> Gain14/1
  Demux/4 -> Gain15/1
  [Xg] -> Gain4/1
  [Yg] -> Gain5/1
  [beta] -> Gain/1
  [vx_vehicle] -> Gain1/1
  [vy_vehicle] -> Gain2/1
  [yawRate_vehicle] -> Gain3/1
  Gain/1 -> Mux/10
  Gain7/1 -> Mux/1, Add/1
  Gain6/1 -> Mux/2, Add/2
  Gain8/1 -> Mux/3, Add1/1
  Gain9/1 -> Mux/8, Add1/2
  Gain10/1 -> Mux/9, Add2/1
  Gain11/1 -> Mux/11, Add2/2
  Gain12/1 -> Mux/4
  Gain13/1 -> Mux/5
  Gain14/1 -> Mux/6
  Gain15/1 -> Mux/7

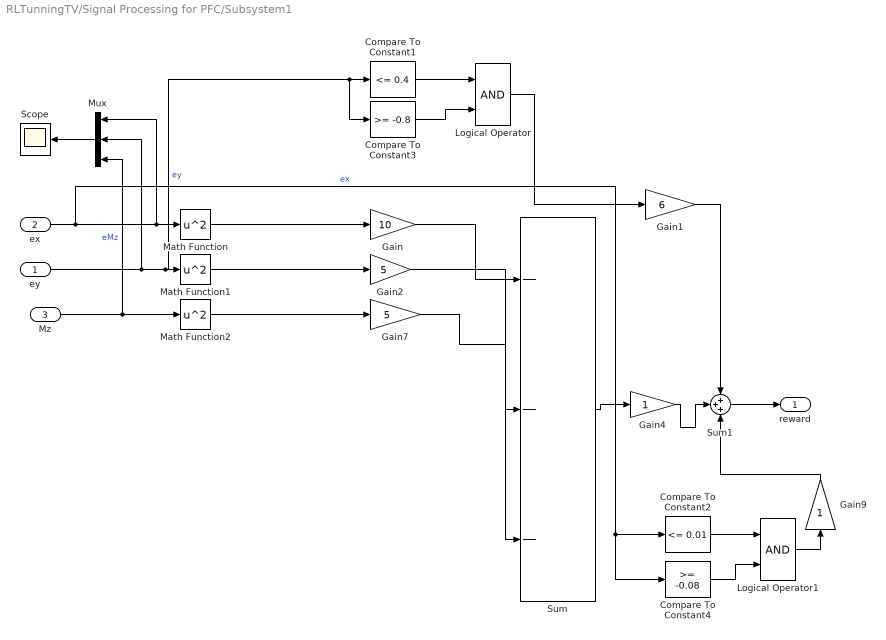
== system RLTunningTV/Signal Processing for PFC/Subsystem1 ==
  ey : Inport
  ex : Inport  Port=2
  Mz : Inport  Port=3
  Compare To Constant1 : simulink/Logic and Bit Operations/Compare To Constant  relop=<=  const=0.4  OutDataTypeStr=boolean
  Compare To Constant2 : simulink/Logic and Bit Operations/Compare To Constant  relop=<=  const=0.01  OutDataTypeStr=boolean
  Compare To Constant3 : simulink/Logic and Bit Operations/Compare To Constant  relop=>=  const=-0.8  OutDataTypeStr=boolean
  Compare To Constant4 : simulink/Logic and Bit Operations/Compare To Constant  relop=>=  const=-0.08  OutDataTypeStr=boolean
  Gain : Gain  Gain=10
  Gain1 : Gain  Gain=6
  Gain2 : Gain  Gain=5
  Gain4 : Gain
  Gain7 : Gain  Gain=5
  Gain9 : Gain
  Logical Operator : Logic  AllPortsSameDT=off  OutDataTypeStr=boolean
  Logical Operator1 : Logic  AllPortsSameDT=off  OutDataTypeStr=boolean
  Math Function : Math  Operator=square  SignedPower=off  SaturateOnIntegerOverflow=on
  Math Function1 : Math  Operator=square  SignedPower=off  SaturateOnIntegerOverflow=on
  Math Function2 : Math  Operator=square  SignedPower=off  SaturateOnIntegerOverflow=on
  Mux : Mux  Inputs=3
  Scope : Scope
  Sum : Sum  Inputs=---
  Sum1 : Sum  Inputs=+++
  reward : Outport  VectorParamsAs1DForOutWhenUnconnected=off
  wires:
  Gain/1 -> Sum/1
  Gain7/1 -> Sum/3
  Gain2/1 -> Sum/2
  Sum/1 -> Gain4/1
  Gain4/1 -> Sum1/2
  Logical Operator/1 -> Gain1/1
  Gain1/1 -> Sum1/1
  Compare To Constant1/1 -> Logical Operator/1
  Compare To Constant3/1 -> Logical Operator/2
  Compare To Constant2/1 -> Logical Operator1/1
  Compare To Constant4/1 -> Logical Operator1/2
  Logical Operator1/1 -> Gain9/1
  Gain9/1 -> Sum1/3
  Mux/1 -> Scope/1
  ex/1 -> Compare To Constant2/1, Compare To Constant4/1, Mux/1, Math Function/1  "ex"
  ey/1 -> Mux/2, Compare To Constant3/1, Compare To Constant1/1, Math Function1/1  "ey"
  Mz/1 -> Mux/3, Math Function2/1  "eMz"
  Math Function/1 -> Gain/1
  Math Function1/1 -> Gain2/1
  Math Function2/1 -> Gain7/1
  Sum1/1 -> reward/1

== system RLTunningTV/Signal Processing for PFC/Subsystem2 ==
  ex : Inport
  ey : Inport  Port=2
  Mz : Inport  Port=3
  Lateral deviation : simulink/Logic and Bit Operations/Compare To Constant  relop=>  const=10000  OutDataTypeStr=boolean
  Lateral deviation1 : simulink/Logic and Bit Operations/Compare To Constant  relop=<=  const=-0.3  OutDataTypeStr=boolean
  Lateral deviation2 : simulink/Logic and Bit Operations/Compare To Constant  relop=>=  const=0.3  OutDataTypeStr=boolean
  Logical Operator : Logic  Operator=OR  Inputs=5  AllPortsSameDT=off  OutDataTypeStr=boolean
  Relative Distance : simulink/Logic and Bit Operations/Compare To Constant  relop=>  const=10000  OutDataTypeStr=boolean
  Velocity : simulink/Logic and Bit Operations/Compare To Constant  relop=>  const=10000  OutDataTypeStr=boolean
  isDone : Outport  VectorParamsAs1DForOutWhenUnconnected=off
  wires:
  Velocity/1 -> Logical Operator/2
  Relative Distance/1 -> Logical Operator/1
  ex/1 -> Relative Distance/1
  Logical Operator/1 -> isDone/1
  ey/1 -> Velocity/1
  Mz/1 -> Lateral deviation/1
  Lateral deviation/1 -> Logical Operator/3
  [beta] -> Lateral deviation2/1, Lateral deviation1/1
  Lateral deviation1/1 -> Logical Operator/4
  Lateral deviation2/1 -> Logical Operator/5

== system RLTunningTV/Environment/DCIM/Tire_model ==
  "slip " : Inport
  alpha : Inport  Port=2
  Constant1 : Constant  Value=lr*(M*g)/(2*(lr+lf))
  Constant4 : Constant  Value=lf*(M*g)/(2*(lr+lf))
  Demux : Demux
  Demux1 : Demux
  Pacejka_Fx : MATLAB Function  TreatAsAtomicUnit=on
  Pacejka_Fy : MATLAB Function  TreatAsAtomicUnit=on
  Fx [N] : Outport  VectorParamsAs1DForOutWhenUnconnected=off
  Fy [N] : Outport  Port=2  VectorParamsAs1DForOutWhenUnconnected=off
  wires:
  Constant4/1 -> Pacejka_Fy/7(Fz_RR), Pacejka_Fy/8(Fz_RL), Pacejka_Fx/8(Fz_RL), Pacejka_Fx/7(Fz_RR)
  Constant1/1 -> Pacejka_Fx/5(Fz_FR), Pacejka_Fy/5(Fz_FR), Pacejka_Fx/6(Fz_FL), Pacejka_Fy/6(Fz_FL)
  "slip "/1 -> Demux/1
  Pacejka_Fy/1(Fy) -> Fy [N]/1
  Pacejka_Fx/1(Fx) -> Fx [N]/1
  Demux/2 -> Pacejka_Fx/2(slip_FL)
  Demux/3 -> Pacejka_Fx/3(slip_RR)
  Demux/1 -> Pacejka_Fx/1(slip_FR)  "slip_FR_vehicle"
  Demux/4 -> Pacejka_Fx/4(slip_RL)
  alpha/1 -> Demux1/1
  Demux1/1 -> Pacejka_Fy/1(alphaFR)
  Demux1/2 -> Pacejka_Fy/2(alphaFL)
  Demux1/3 -> Pacejka_Fy/3(alphaRR)
  Demux1/4 -> Pacejka_Fy/4(alphaRL)

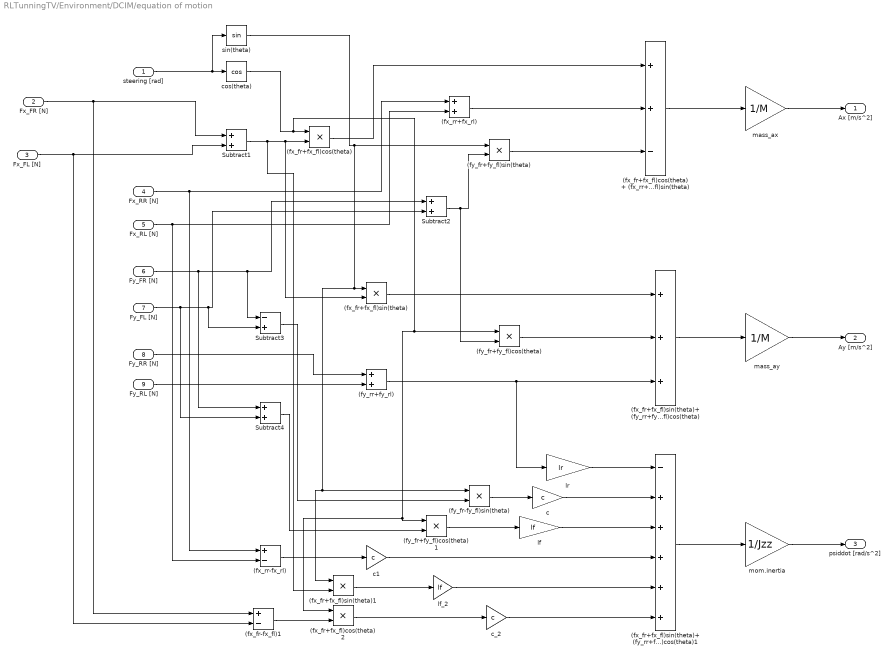
== system RLTunningTV/Environment/DCIM/equation of motion ==
  steering [rad] : Inport
  Fx_FR [N] : Inport  Port=2
  Fx_FL [N] : Inport  Port=3
  Fx_RR [N] : Inport  Port=4
  Fx_RL [N] : Inport  Port=5
  Fy_FR [N] : Inport  Port=6
  Fy_FL [N] : Inport  Port=7
  Fy_RR [N] : Inport  Port=8
  Fy_RL [N] : Inport  Port=9
  (fx_fr+fx_fl)cos(theta) : Product
  (fx_fr+fx_fl)cos(theta)+ (fx_rr+fx_rl)- (fy_fr+fy_fl)sin(theta) : Sum  Inputs=++-
  (fx_fr+fx_fl)cos(theta)2 : Product
  (fx_fr+fx_fl)sin(theta) : Product
  (fx_fr+fx_fl)sin(theta)+ (fy_rr+fy_rl)+ (fy_fr+fy_fl)cos(theta) : Sum  Inputs=+++
  (fx_fr+fx_fl)sin(theta)+ (fy_rr+fy_rl)+ (fy_fr+fy_fl)cos(theta)1 : Sum  Inputs=-+++++
  (fx_fr+fx_fl)sin(theta)1 : Product
  (fx_fr-fx_fl)1 : Sum  Inputs=+-
  (fx_rr+fx_rl) : Sum
  (fx_rr-fx_rl) : Sum  Inputs=+-
  (fy_fr+fy_fl)cos(theta) : Product
  (fy_fr+fy_fl)cos(theta)1 : Product
  (fy_fr+fy_fl)sin(theta) : Product
  (fy_fr-fy_fl)sin(theta) : Product
  (fy_rr+fy_rl) : Sum
  Subtract1 : Sum
  Subtract2 : Sum
  Subtract3 : Sum  Inputs=-+
  Subtract4 : Sum
  c : Gain  Gain=c
  c1 : Gain  Gain=c
  "c_2 " : Gain  Gain=c
  "cos(theta) " : Trigonometry  Operator=cos
  lf : Gain  Gain=lf
  lf_2 : Gain  Gain=lf
  lr : Gain  Gain=lr
  mass_ax : Gain  Gain=1/M
  mass_ay : Gain  Gain=1/M
  mom.inertia : Gain  Gain=1/Jzz
  "sin(theta) " : Trigonometry
  Ax [m/s^2] : Outport  VectorParamsAs1DForOutWhenUnconnected=off
  Ay [m/s^2] : Outport  Port=2  VectorParamsAs1DForOutWhenUnconnected=off
  psiddot [rad/s^2] : Outport  Port=3  VectorParamsAs1DForOutWhenUnconnected=off
  wires:
  Fx_FL [N]/1 -> (fx_fr-fx_fl)1/2, Subtract1/2
  Fx_FR [N]/1 -> (fx_fr-fx_fl)1/1, Subtract1/1
  Subtract1/1 -> (fx_fr+fx_fl)sin(theta)1/2, (fx_fr+fx_fl)sin(theta)/2, (fx_fr+fx_fl)cos(theta)/2
  steering [rad]/1 -> "sin(theta) "/1, "cos(theta) "/1
  "cos(theta) "/1 -> (fy_fr+fy_fl)cos(theta)/1, (fx_fr+fx_fl)cos(theta)2/1, (fy_fr+fy_fl)cos(theta)1/1, (fx_fr+fx_fl)cos(theta)/1
  (fx_fr+fx_fl)cos(theta)+ (fx_rr+fx_rl)- (fy_fr+fy_fl)sin(theta)/1 -> mass_ax/1
  mass_ax/1 -> Ax [m/s^2]/1
  (fx_fr+fx_fl)cos(theta)/1 -> (fx_fr+fx_fl)cos(theta)+ (fx_rr+fx_rl)- (fy_fr+fy_fl)sin(theta)/1
  Fx_RR [N]/1 -> (fx_rr-fx_rl)/1, (fx_rr+fx_rl)/1
  Fx_RL [N]/1 -> (fx_rr-fx_rl)/2, (fx_rr+fx_rl)/2
  (fx_rr+fx_rl)/1 -> (fx_fr+fx_fl)cos(theta)+ (fx_rr+fx_rl)- (fy_fr+fy_fl)sin(theta)/2
  "sin(theta) "/1 -> (fy_fr-fy_fl)sin(theta)/1, (fx_fr+fx_fl)sin(theta)1/1, (fx_fr+fx_fl)sin(theta)/1, (fy_fr+fy_fl)sin(theta)/1
  Subtract2/1 -> (fy_fr+fy_fl)cos(theta)/2, (fy_fr+fy_fl)sin(theta)/2
  Fy_FR [N]/1 -> Subtract4/1, Subtract3/1, Subtract2/1
  Fy_FL [N]/1 -> Subtract4/2, Subtract3/2, Subtract2/2
  (fy_fr+fy_fl)sin(theta)/1 -> (fx_fr+fx_fl)cos(theta)+ (fx_rr+fx_rl)- (fy_fr+fy_fl)sin(theta)/3
  (fx_fr+fx_fl)sin(theta)+ (fy_rr+fy_rl)+ (fy_fr+fy_fl)cos(theta)/1 -> mass_ay/1
  mass_ay/1 -> Ay [m/s^2]/1
  (fx_fr+fx_fl)sin(theta)/1 -> (fx_fr+fx_fl)sin(theta)+ (fy_rr+fy_rl)+ (fy_fr+fy_fl)cos(theta)/1
  (fy_fr+fy_fl)cos(theta)/1 -> (fx_fr+fx_fl)sin(theta)+ (fy_rr+fy_rl)+ (fy_fr+fy_fl)cos(theta)/2
  Fy_RR [N]/1 -> (fy_rr+fy_rl)/1
  Fy_RL [N]/1 -> (fy_rr+fy_rl)/2
  (fy_rr+fy_rl)/1 -> lr/1, (fx_fr+fx_fl)sin(theta)+ (fy_rr+fy_rl)+ (fy_fr+fy_fl)cos(theta)/3
  mom.inertia/1 -> psiddot [rad/s^2]/1
  (fx_fr+fx_fl)sin(theta)+ (fy_rr+fy_rl)+ (fy_fr+fy_fl)cos(theta)1/1 -> mom.inertia/1
  lr/1 -> (fx_fr+fx_fl)sin(theta)+ (fy_rr+fy_rl)+ (fy_fr+fy_fl)cos(theta)1/1
  c/1 -> (fx_fr+fx_fl)sin(theta)+ (fy_rr+fy_rl)+ (fy_fr+fy_fl)cos(theta)1/2
  (fy_fr-fy_fl)sin(theta)/1 -> c/1
  Subtract3/1 -> (fy_fr-fy_fl)sin(theta)/2
  lf/1 -> (fx_fr+fx_fl)sin(theta)+ (fy_rr+fy_rl)+ (fy_fr+fy_fl)cos(theta)1/3
  (fy_fr+fy_fl)cos(theta)1/1 -> lf/1
  Subtract4/1 -> (fy_fr+fy_fl)cos(theta)1/2
  (fx_rr-fx_rl)/1 -> c1/1
  c1/1 -> (fx_fr+fx_fl)sin(theta)+ (fy_rr+fy_rl)+ (fy_fr+fy_fl)cos(theta)1/4
  lf_2/1 -> (fx_fr+fx_fl)sin(theta)+ (fy_rr+fy_rl)+ (fy_fr+fy_fl)cos(theta)1/5
  (fx_fr+fx_fl)sin(theta)1/1 -> lf_2/1
  "c_2 "/1 -> (fx_fr+fx_fl)sin(theta)+ (fy_rr+fy_rl)+ (fy_fr+fy_fl)cos(theta)1/6
  (fx_fr+fx_fl)cos(theta)2/1 -> "c_2 "/1
  (fx_fr-fx_fl)1/1 -> (fx_fr+fx_fl)cos(theta)2/2

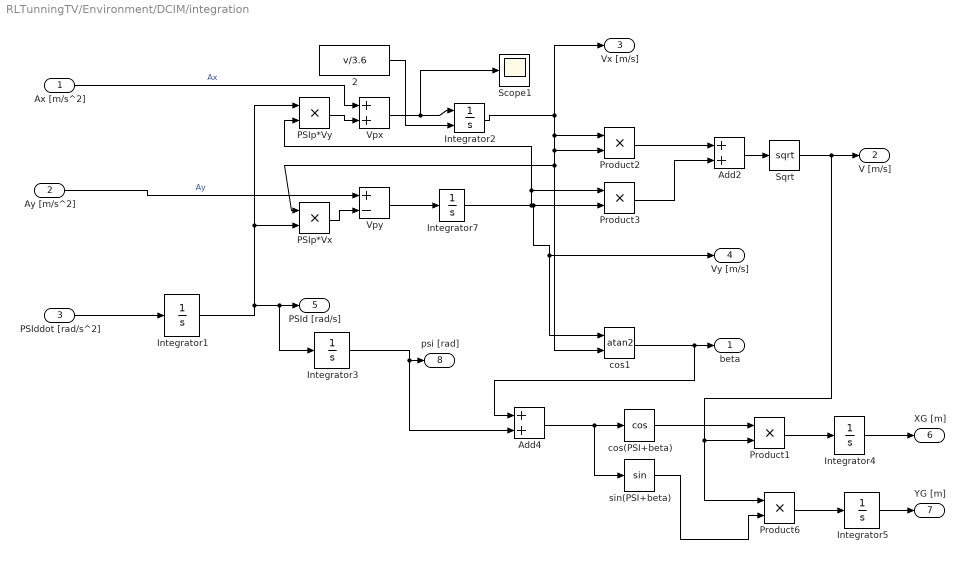
== system RLTunningTV/Environment/DCIM/integration ==
  Ax [m/s^2] : Inport
  Ay [m/s^2] : Inport  Port=2
  PSIddot [rad/s^2] : Inport  Port=3
  2 : Constant  Value=v/3.6
  Add2 : Sum
  Add4 : Sum
  Integrator{1,3..5,7} (5 alike) : Integrator
  Integrator2 : Integrator  InitialConditionSource=external  InitialCondition=v/3.6
  PSIp*Vx : Product  RndMeth=Zero
  PSIp*Vy : Product  RndMeth=Zero
  Product{1..3,6} (4 alike) : Product  RndMeth=Zero
  Scope1 : Scope
  Sqrt : Sqrt  SaturateOnIntegerOverflow=on
  Vpx : Sum
  Vpy : Sum  Inputs=+-
  cos(PSI+beta) : Trigonometry  Operator=cos
  cos1 : Trigonometry  Operator=atan2
  sin(PSI+beta) : Trigonometry
  beta : Outport  VectorParamsAs1DForOutWhenUnconnected=off
  V [m/s] : Outport  Port=2  VectorParamsAs1DForOutWhenUnconnected=off
  Vx [m/s] : Outport  Port=3  VectorParamsAs1DForOutWhenUnconnected=off
  Vy [m/s] : Outport  Port=4  VectorParamsAs1DForOutWhenUnconnected=off
  PSId [rad/s] : Outport  Port=5  VectorParamsAs1DForOutWhenUnconnected=off
  XG [m] : Outport  Port=6  VectorParamsAs1DForOutWhenUnconnected=off
  YG [m] : Outport  Port=7  VectorParamsAs1DForOutWhenUnconnected=off
  psi [rad] : Outport  Port=8  VectorParamsAs1DForOutWhenUnconnected=off
  wires:
  Integrator1/1 -> Integrator3/1, PSId [rad/s]/1, PSIp*Vy/1, PSIp*Vx/2
  PSIddot [rad/s^2]/1 -> Integrator1/1
  Integrator2/1 -> Product2/1, Product2/2, cos1/2, PSIp*Vx/1, Vx [m/s]/1
  Ax [m/s^2]/1 -> Vpx/1  "Ax"
  PSIp*Vy/1 -> Vpx/2
  PSIp*Vx/1 -> Vpy/2
  Vpy/1 -> Integrator7/1
  Integrator7/1 -> Product3/1, PSIp*Vy/2, Vy [m/s]/1, cos1/1, Product3/2
  Ay [m/s^2]/1 -> Vpy/1  "Ay"
  cos1/1 -> beta/1, Add4/1
  Product2/1 -> Add2/1
  Product3/1 -> Add2/2
  Add2/1 -> Sqrt/1
  Sqrt/1 -> V [m/s]/1, Product1/2, Product6/1
  Integrator3/1 -> Add4/2, psi [rad]/1
  cos(PSI+beta)/1 -> Product1/1
  sin(PSI+beta)/1 -> Product6/2
  Add4/1 -> cos(PSI+beta)/1, sin(PSI+beta)/1
  Product6/1 -> Integrator5/1
  Product1/1 -> Integrator4/1
  Integrator4/1 -> XG [m]/1
  Integrator5/1 -> YG [m]/1
  Vpx/1 -> Scope1/1, Integrator2/1
  2/1 -> Integrator2/2

== system RLTunningTV/Environment/DCIM/lateral slip ==
  steering : Inport
  vx : Inport  Port=2
  vy : Inport  Port=3
  psid : Inport  Port=4
  Mux : Mux
  Scope : Scope
  alpha_FL : Subsystem  TreatAsAtomicUnit=on
  alpha_FR : Subsystem  TreatAsAtomicUnit=on
  alpha_RL : Subsystem  TreatAsAtomicUnit=on
  alpha_RR : Subsystem  TreatAsAtomicUnit=on
  alpha[4x1] : Outport  VectorParamsAs1DForOutWhenUnconnected=off
  wires:
  steering/1 -> alpha_FL/1(steering), alpha_FR/1(steering)
  vx/1 -> alpha_RL/1(vx), alpha_RR/1(vx), alpha_FL/2(vx), alpha_FR/2(vx)
  vy/1 -> alpha_RL/2(vy), alpha_RR/2(vy), alpha_FL/3(vy), alpha_FR/3(vy)
  psid/1 -> alpha_RL/3(psid), alpha_RR/3(psid), alpha_FL/4(psid), alpha_FR/4(psid)
  Mux/1 -> alpha[4x1]/1
  alpha_FR/1(alpha_FR) -> Scope/1, Mux/1
  alpha_FL/1(alpha_FL) -> Mux/2
  alpha_RR/1(alpha_RR) -> Mux/3
  alpha_RL/1(alpha_RL) -> Mux/4

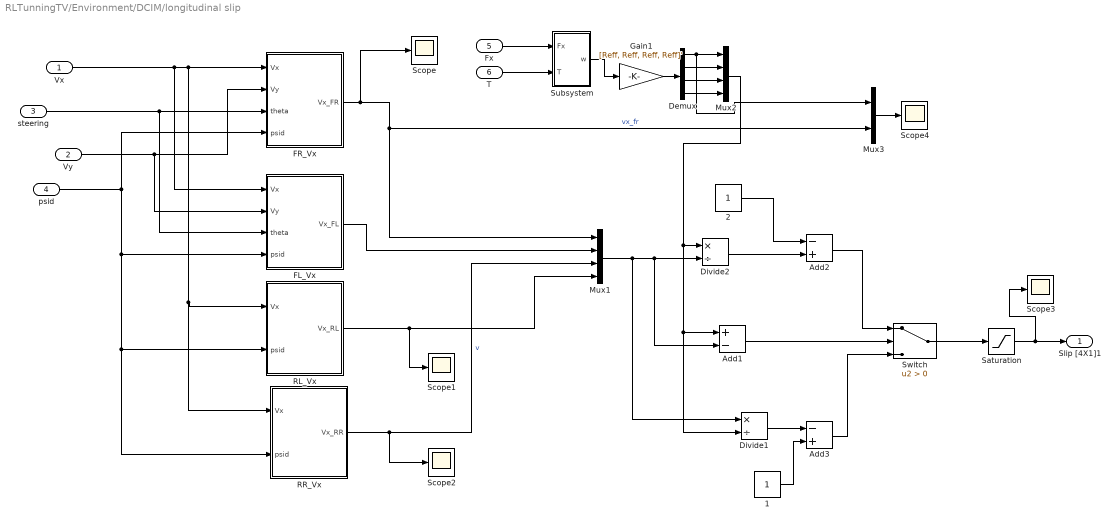
== system RLTunningTV/Environment/DCIM/longitudinal slip ==
  Vx : Inport
  Vy : Inport  Port=2
  steering : Inport  Port=3
  psid : Inport  Port=4
  Fx : Inport  Port=5
  T : Inport  Port=6
  1 : Constant
  2 : Constant
  Add1 : Sum  Inputs=+-
  Add2 : Sum  Inputs=-+
  Add3 : Sum  Inputs=-+
  Demux : Demux
  Divide1 : Product  Inputs=*/
  Divide2 : Product  Inputs=*/
  FL_Vx : Subsystem  TreatAsAtomicUnit=on
  FR_Vx : Subsystem  TreatAsAtomicUnit=on
  Gain1 : Gain  Gain=[Reff, Reff, Reff, Reff]'
  Mux1 : Mux
  Mux2 : Mux
  Mux3 : Mux  Inputs=2
  RL_Vx : Subsystem  TreatAsAtomicUnit=on
  RR_Vx : Subsystem  TreatAsAtomicUnit=on
  Saturation : Saturate  UpperLimit=1  LowerLimit=-1
  Scope{,1..4} (5 alike) : Scope
  Subsystem : Subsystem
  Switch : Switch  Criteria=u2 > Threshold
  Slip [4X1]1 : Outport  VectorParamsAs1DForOutWhenUnconnected=off
  wires:
  Switch/1 -> Saturation/1
  Mux3/1 -> Scope4/1
  Mux2/1 -> Divide2/1, Add1/1, Divide1/2
  Demux/4 -> Mux2/4
  Demux/3 -> Mux2/3
  Demux/2 -> Mux2/2
  Demux/1 -> Mux2/1, Mux3/1
  Saturation/1 -> Slip [4X1]1/1, Scope3/1
  Vx/1 -> FL_Vx/1(Vx), FR_Vx/1(Vx), RR_Vx/1(Vx), RL_Vx/1(Vx)
  psid/1 -> FL_Vx/4(psid), RR_Vx/2(psid), RL_Vx/2(psid), FR_Vx/4(psid)
  Subsystem/1(w) -> Gain1/1
  Vy/1 -> FL_Vx/2(Vy), FR_Vx/2(Vy)
  steering/1 -> FL_Vx/3(theta), FR_Vx/3(theta)
  Divide2/1 -> Add2/2
  2/1 -> Add2/1
  FR_Vx/1(Vx_FR) -> Scope/1, Mux1/1, Mux3/2  "vx_fr"
  FL_Vx/1(Vx_FL) -> Mux1/2
  RR_Vx/1(Vx_RR) -> Scope2/1, Mux1/3  "v"
  RL_Vx/1(Vx_RL) -> Scope1/1, Mux1/4
  Mux1/1 -> Divide1/1, Add1/2, Divide2/2
  Add1/1 -> Switch/2
  Divide1/1 -> Add3/1
  1/1 -> Add3/2
  Add3/1 -> Switch/3
  Add2/1 -> Switch/1
  Gain1/1 -> Demux/1
  Fx/1 -> Subsystem/1(Fx)
  T/1 -> Subsystem/2(T)

== system RLTunningTV/Environment/Vehicle Model/Subsystem ==
  Scope{,1..6} (7 alike) : Scope
  To Workspace : ToWorkspace  VariableName=Xg  SaveFormat=Structure With Time  SampleTime=-1
  To Workspace1 : ToWorkspace  VariableName=Yg  SaveFormat=Structure With Time  SampleTime=-1
  To Workspace2 : ToWorkspace  VariableName=Fx_CG  SaveFormat=Structure With Time  SampleTime=-1
  To Workspace3 : ToWorkspace  VariableName=Fy_CG  SaveFormat=Structure With Time  SampleTime=-1
  To Workspace4 : ToWorkspace  VariableName=Mz_CG  SaveFormat=Structure With Time  SampleTime=-1
  To Workspace5 : ToWorkspace  VariableName=Ax  SaveFormat=Structure With Time  SampleTime=-1
  To Workspace6 : ToWorkspace  VariableName=Ay  SaveFormat=Structure With Time  SampleTime=-1
  wires:
  [Xg] -> To Workspace/1, Scope/1
  [Fx_CG] -> To Workspace2/1, Scope2/1
  [Fy_CG] -> To Workspace3/1, Scope3/1
  [Mz_CG] -> To Workspace4/1, Scope4/1
  [Yg] -> To Workspace1/1, Scope1/1
  [Ax] -> To Workspace5/1, Scope5/1
  [Ay] -> Scope6/1, To Workspace6/1

== system RLTunningTV/Environment/Vehicle Model/Tire_model ==
  "slip " : Inport
  alpha : Inport  Port=2
  Constant : Constant  Value=LMUX
  Constant1 : Constant  Value=lr*(M*g)/(2*(lr+lf))
  Constant2 : Constant  Value=LMUY
  Constant4 : Constant  Value=lf*(M*g)/(2*(lr+lf))
  Demux : Demux
  Demux1 : Demux
  Display : Display
  Display1 : Display
  Mux : Mux
  Pacejka_Fx : MATLAB Function  TreatAsAtomicUnit=on
  Pacejka_Fy : MATLAB Function  TreatAsAtomicUnit=on
  Fx [N] : Outport  VectorParamsAs1DForOutWhenUnconnected=off
  Fy [N] : Outport  Port=2  VectorParamsAs1DForOutWhenUnconnected=off
  mux : Outport  Port=3  VectorParamsAs1DForOutWhenUnconnected=off
  muy : Outport  Port=4  VectorParamsAs1DForOutWhenUnconnected=off
  Fz : Outport  Port=5  VectorParamsAs1DForOutWhenUnconnected=off
  wires:
  Demux1/4 -> Pacejka_Fy/4(alphaRL)
  Demux1/3 -> Pacejka_Fy/3(alphaRR)
  Demux1/2 -> Pacejka_Fy/2(alphaFL)
  Demux1/1 -> Pacejka_Fy/1(alphaFR)
  alpha/1 -> Demux1/1
  Demux/4 -> Pacejka_Fx/4(slip_RL)
  Demux/1 -> Pacejka_Fx/1(slip_FR)  "slip_FR_vehicle"
  Demux/3 -> Pacejka_Fx/3(slip_RR)
  Demux/2 -> Pacejka_Fx/2(slip_FL)
  Pacejka_Fx/1(Fx) -> Fx [N]/1
  Pacejka_Fy/1(Fy) -> Fy [N]/1
  Pacejka_Fx/2(mux) -> Display/1, mux/1
  Pacejka_Fy/2(muy) -> Display1/1, muy/1
  "slip "/1 -> Demux/1
  Constant1/1 -> Pacejka_Fy/6(Fz_FL), Pacejka_Fx/6(Fz_FL), Pacejka_Fy/5(Fz_FR), Pacejka_Fx/5(Fz_FR), Mux/2, Mux/1
  Constant4/1 -> Mux/4, Mux/3, Pacejka_Fx/7(Fz_RR), Pacejka_Fx/8(Fz_RL), Pacejka_Fy/8(Fz_RL), Pacejka_Fy/7(Fz_RR)
  Mux/1 -> Fz/1
  Constant/1 -> Pacejka_Fx/9(LMUX)
  Constant2/1 -> Pacejka_Fy/9(LMUY)

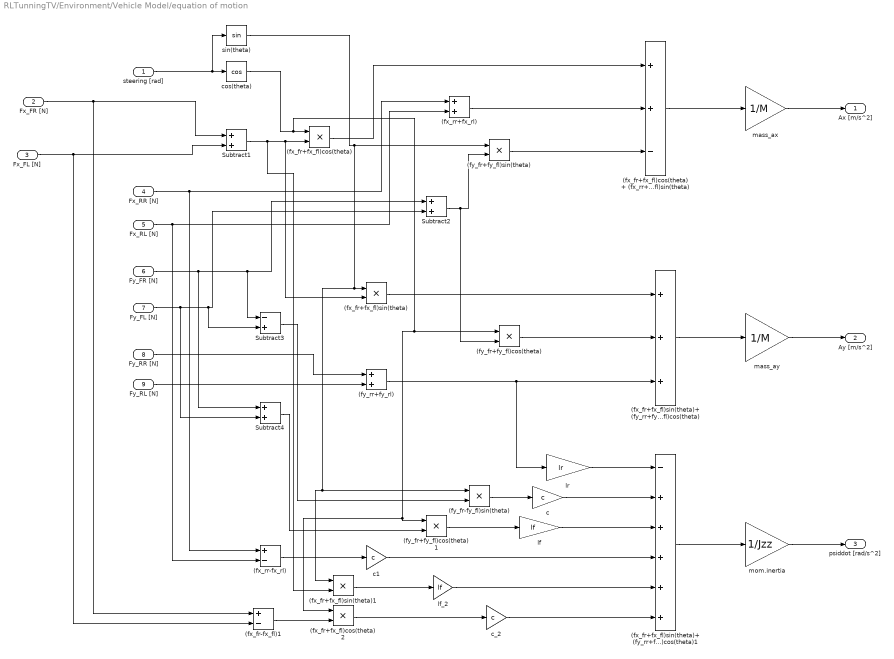
== system RLTunningTV/Environment/Vehicle Model/equation of motion ==
  steering [rad] : Inport
  Fx_FR [N] : Inport  Port=2
  Fx_FL [N] : Inport  Port=3
  Fx_RR [N] : Inport  Port=4
  Fx_RL [N] : Inport  Port=5
  Fy_FR [N] : Inport  Port=6
  Fy_FL [N] : Inport  Port=7
  Fy_RR [N] : Inport  Port=8
  Fy_RL [N] : Inport  Port=9
  (fx_fr+fx_fl)cos(theta) : Product
  (fx_fr+fx_fl)cos(theta)+ (fx_rr+fx_rl)- (fy_fr+fy_fl)sin(theta) : Sum  Inputs=++-
  (fx_fr+fx_fl)cos(theta)2 : Product
  (fx_fr+fx_fl)sin(theta) : Product
  (fx_fr+fx_fl)sin(theta)+ (fy_rr+fy_rl)+ (fy_fr+fy_fl)cos(theta) : Sum  Inputs=+++
  (fx_fr+fx_fl)sin(theta)+ (fy_rr+fy_rl)+ (fy_fr+fy_fl)cos(theta)1 : Sum  Inputs=-+++++
  (fx_fr+fx_fl)sin(theta)1 : Product
  (fx_fr-fx_fl)1 : Sum  Inputs=+-
  (fx_rr+fx_rl) : Sum
  (fx_rr-fx_rl) : Sum  Inputs=+-
  (fy_fr+fy_fl)cos(theta) : Product
  (fy_fr+fy_fl)cos(theta)1 : Product
  (fy_fr+fy_fl)sin(theta) : Product
  (fy_fr-fy_fl)sin(theta) : Product
  (fy_rr+fy_rl) : Sum
  Subtract1 : Sum
  Subtract2 : Sum
  Subtract3 : Sum  Inputs=-+
  Subtract4 : Sum
  c : Gain  Gain=c
  c1 : Gain  Gain=c
  "c_2 " : Gain  Gain=c
  "cos(theta) " : Trigonometry  Operator=cos
  lf : Gain  Gain=lf
  lf_2 : Gain  Gain=lf
  lr : Gain  Gain=lr
  mass_ax : Gain  Gain=1/M
  mass_ay : Gain  Gain=1/M
  mom.inertia : Gain  Gain=1/Jzz
  "sin(theta) " : Trigonometry
  Ax [m/s^2] : Outport  VectorParamsAs1DForOutWhenUnconnected=off
  Ay [m/s^2] : Outport  Port=2  VectorParamsAs1DForOutWhenUnconnected=off
  psiddot [rad/s^2] : Outport  Port=3  VectorParamsAs1DForOutWhenUnconnected=off
  wires:
  (fx_fr-fx_fl)1/1 -> (fx_fr+fx_fl)cos(theta)2/2
  (fx_fr+fx_fl)cos(theta)2/1 -> "c_2 "/1
  "c_2 "/1 -> (fx_fr+fx_fl)sin(theta)+ (fy_rr+fy_rl)+ (fy_fr+fy_fl)cos(theta)1/6
  (fx_fr+fx_fl)sin(theta)1/1 -> lf_2/1
  lf_2/1 -> (fx_fr+fx_fl)sin(theta)+ (fy_rr+fy_rl)+ (fy_fr+fy_fl)cos(theta)1/5
  c1/1 -> (fx_fr+fx_fl)sin(theta)+ (fy_rr+fy_rl)+ (fy_fr+fy_fl)cos(theta)1/4
  (fx_rr-fx_rl)/1 -> c1/1
  Subtract4/1 -> (fy_fr+fy_fl)cos(theta)1/2
  (fy_fr+fy_fl)cos(theta)1/1 -> lf/1
  lf/1 -> (fx_fr+fx_fl)sin(theta)+ (fy_rr+fy_rl)+ (fy_fr+fy_fl)cos(theta)1/3
  Subtract3/1 -> (fy_fr-fy_fl)sin(theta)/2
  (fy_fr-fy_fl)sin(theta)/1 -> c/1
  c/1 -> (fx_fr+fx_fl)sin(theta)+ (fy_rr+fy_rl)+ (fy_fr+fy_fl)cos(theta)1/2
  lr/1 -> (fx_fr+fx_fl)sin(theta)+ (fy_rr+fy_rl)+ (fy_fr+fy_fl)cos(theta)1/1
  (fx_fr+fx_fl)sin(theta)+ (fy_rr+fy_rl)+ (fy_fr+fy_fl)cos(theta)1/1 -> mom.inertia/1
  mom.inertia/1 -> psiddot [rad/s^2]/1
  (fy_rr+fy_rl)/1 -> (fx_fr+fx_fl)sin(theta)+ (fy_rr+fy_rl)+ (fy_fr+fy_fl)cos(theta)/3, lr/1
  Fy_RL [N]/1 -> (fy_rr+fy_rl)/2
  Fy_RR [N]/1 -> (fy_rr+fy_rl)/1
  (fy_fr+fy_fl)cos(theta)/1 -> (fx_fr+fx_fl)sin(theta)+ (fy_rr+fy_rl)+ (fy_fr+fy_fl)cos(theta)/2
  (fx_fr+fx_fl)sin(theta)/1 -> (fx_fr+fx_fl)sin(theta)+ (fy_rr+fy_rl)+ (fy_fr+fy_fl)cos(theta)/1
  mass_ay/1 -> Ay [m/s^2]/1
  (fx_fr+fx_fl)sin(theta)+ (fy_rr+fy_rl)+ (fy_fr+fy_fl)cos(theta)/1 -> mass_ay/1
  (fy_fr+fy_fl)sin(theta)/1 -> (fx_fr+fx_fl)cos(theta)+ (fx_rr+fx_rl)- (fy_fr+fy_fl)sin(theta)/3
  Fy_FL [N]/1 -> Subtract2/2, Subtract3/2, Subtract4/2
  Fy_FR [N]/1 -> Subtract2/1, Subtract3/1, Subtract4/1
  Subtract2/1 -> (fy_fr+fy_fl)sin(theta)/2, (fy_fr+fy_fl)cos(theta)/2
  "sin(theta) "/1 -> (fy_fr+fy_fl)sin(theta)/1, (fx_fr+fx_fl)sin(theta)/1, (fx_fr+fx_fl)sin(theta)1/1, (fy_fr-fy_fl)sin(theta)/1
  (fx_rr+fx_rl)/1 -> (fx_fr+fx_fl)cos(theta)+ (fx_rr+fx_rl)- (fy_fr+fy_fl)sin(theta)/2
  Fx_RL [N]/1 -> (fx_rr+fx_rl)/2, (fx_rr-fx_rl)/2
  Fx_RR [N]/1 -> (fx_rr+fx_rl)/1, (fx_rr-fx_rl)/1
  (fx_fr+fx_fl)cos(theta)/1 -> (fx_fr+fx_fl)cos(theta)+ (fx_rr+fx_rl)- (fy_fr+fy_fl)sin(theta)/1
  mass_ax/1 -> Ax [m/s^2]/1
  (fx_fr+fx_fl)cos(theta)+ (fx_rr+fx_rl)- (fy_fr+fy_fl)sin(theta)/1 -> mass_ax/1
  "cos(theta) "/1 -> (fx_fr+fx_fl)cos(theta)/1, (fy_fr+fy_fl)cos(theta)1/1, (fx_fr+fx_fl)cos(theta)2/1, (fy_fr+fy_fl)cos(theta)/1
  steering [rad]/1 -> "cos(theta) "/1, "sin(theta) "/1
  Subtract1/1 -> (fx_fr+fx_fl)cos(theta)/2, (fx_fr+fx_fl)sin(theta)/2, (fx_fr+fx_fl)sin(theta)1/2
  Fx_FR [N]/1 -> Subtract1/1, (fx_fr-fx_fl)1/1
  Fx_FL [N]/1 -> Subtract1/2, (fx_fr-fx_fl)1/2
